simulink model "preg2_simu"  (R2021a)
settings: Solver=VariableStepAuto  StartTime=0.0  StopTime=50  RelTol=1e-3
values from neighbouring files (symbols this model uses):
  Gc = Kp*(1+Td*s)    [preg1.m]    (also in preg2.m = 4.3694)
  sys = 1/(s*s +2*s)    [preg1.m]    (also in preg2.m = 44.4/(0.015*s+1)/100/s)
settings Model: Creator=pierr  LastModifiedBy=pierr

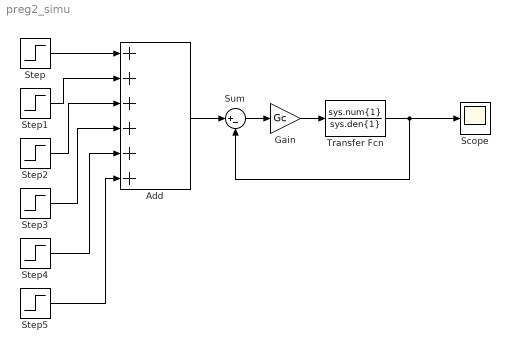
== system preg2_simu ==
  Add : Sum  Inputs=++++++
  Gain : Gain  Gain=Gc
  Scope : Scope
  Step : Step  Time=0  After=pi  SampleTime=0
  Step1 : Step  Time=8  After=pi  SampleTime=0
  Step2 : Step  Time=16  After=pi  SampleTime=0
  Step3 : Step  Time=24  After=pi  SampleTime=0
  Step4 : Step  Time=32  After=pi  SampleTime=0
  Step5 : Step  Time=40  After=pi  SampleTime=0
  Sum : Sum  Inputs=|+-
  Transfer Fcn : TransferFcn  Numerator=sys.num{1}  Denominator=sys.den{1}
  wires:
  Step/1 -> Add/1
  Step1/1 -> Add/2
  Step2/1 -> Add/3
  Step3/1 -> Add/4
  Step4/1 -> Add/5
  Step5/1 -> Add/6
  Add/1 -> Sum/1
  Sum/1 -> Gain/1
  Gain/1 -> Transfer Fcn/1
  Transfer Fcn/1 -> Scope/1, Sum/2
